simulink model "msk_ref"  (Simulink 7.9)
settings: Solver=FixedStepDiscrete  SolverMode=SingleTasking  StartTime=0.0  StopTime=1e4  RelTol=1e-3
model workspace (MATLAB code in the model file):
  | N = 14; % Oversampling factor
  | traceback_depth = 16; % Traceback depth
  | Tsym = 1/280000;
undefined symbols (not defined in the file or in its folder): get
libraries: commsink2 x2, commdigbbndcpm2 x2, commchan3 x1, commrandsrc2 x1
settings Model: Creator=sszilvasi  LastModifiedBy=sszilvasi
settings DataIOCC: SaveOutput=off  SignalLogging=off  SaveTime=off
settings OptimizationCC: InlineParams=on
settings DebuggingCC: AlgebraicLoopMsg=error

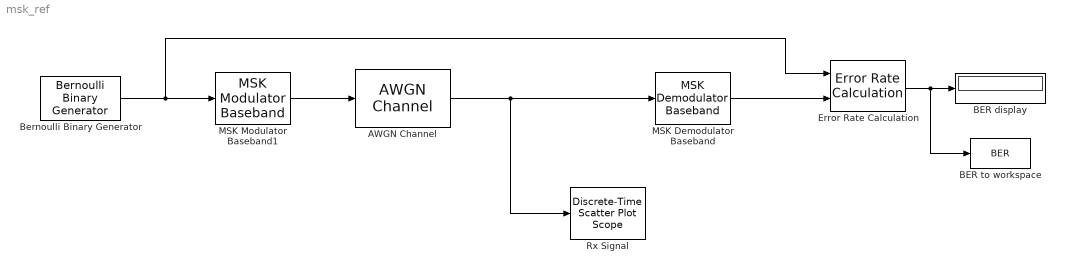
== system msk_ref ==
  AWGN Channel : commchan3/AWGN Channel  InputProcessing=Columns as channels (frame based)  seed=67  noiseMode="Signal to noise ratio  (Eb/No)"  EbNodB=40  EsNodB=10  SNRdB=10  bitsPerSym=1  Ps=1  Tsym=1  variance=1
  BER display : Display
  BER to workspace : ToWorkspace  VariableName=BER  SampleTime=-1  SaveFormat=Timeseries
  Bernoulli Binary Generator : commrandsrc2/Bernoulli Binary Generator  P=0.5  seed=61  Ts=1  frameBased=on  sampPerFrame=100  orient=off  outDataType=double
  Error Rate Calculation : commsink2/Error Rate Calculation  N=traceback_depth % Traceback depth plus timing recovery delay  st_delay=0  cp_mode=Entire frame  subframe=[]  PMode=Port  WsName=ErrorVec  RsMode2=off  stop=off  numErr=100  maxBits=1e6
  MSK Demodulator Baseband : commdigbbndcpm2/MSK Demodulator Baseband  outputType=Bit  phaseOffset=0  samplesPerSymbol=N  RateOptions=Enforce single-rate processing  traceBack=traceback_depth  outDType=double
  MSK Modulator Baseband1 : commdigbbndcpm2/MSK Modulator Baseband  inputType=Bit  phaseOffset=0  samplesPerSymbol=N  RateOptions=Enforce single-rate processing  outDataType=double
  Rx Signal : commsink2/Discrete-Time Scatter Plot Scope  Tag=ScatterPlot  sampPerSymb=1  offsetEye=0  numTraces=40  numNewFrames=40  LineMarkers=.  LineColors=b  fading=on  render=on  AxisGrid=on  xMin=-3.3  xMax=3.315  yMin=-3.3  yMax=3.315  inphaseLabel=In-phase Amplitude  quadratureLabel=Quadrature Amplitude  openScopeAtSimStart=off  FrameNumber=off  FigPos=get(0,'defaultfigureposition');  figTitle=Scatter Plot  numLinesMax=8  block_type_=scatter
  wires:
  Bernoulli Binary Generator/1 -> Error Rate Calculation/1, MSK Modulator Baseband1/1
  MSK Modulator Baseband1/1 -> AWGN Channel/1
  AWGN Channel/1 -> Rx Signal/1, MSK Demodulator Baseband/1
  MSK Demodulator Baseband/1 -> Error Rate Calculation/2
  Error Rate Calculation/1 -> BER display/1, BER to workspace/1
